simulink model "Follower_V2V"  (R2014b)
settings: Solver=ode3  SolverMode=SingleTasking  StartTime=0.0  StopTime=10.0  FixedStep=sampleTimes.main  RelTol=1e-3
model workspace (MAT data in the model file):
  spacing = 0
  vehicle = 0
undefined symbols (not defined in the file or in its folder): delays, sampleTimes
libraries: simulink x15
settings Model: ParameterArgumentNames=vehicle,spacing  Creator=uos  LastModifiedBy=uos

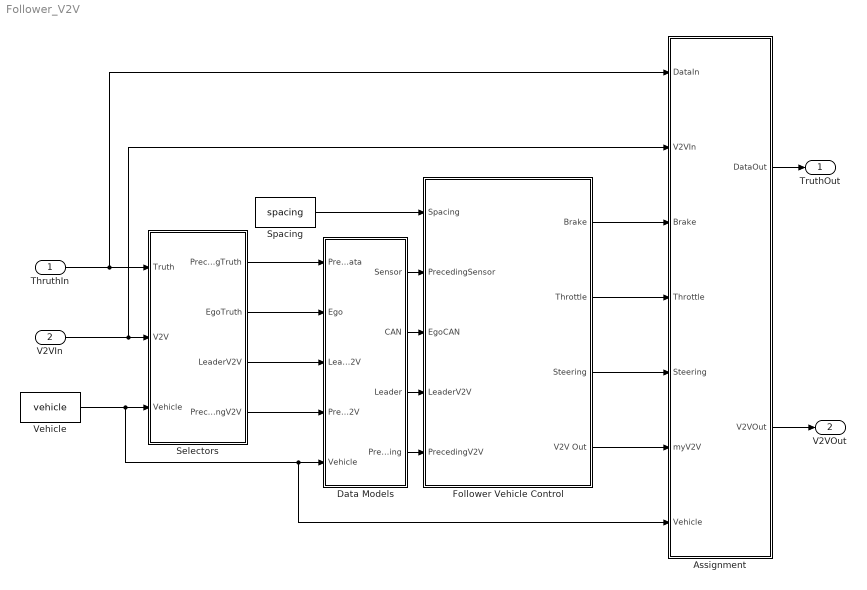
== system Follower_V2V ==
  ThruthIn : Inport  OutDataTypeStr=Bus: VehicleBus  PortDimensions=10  BusOutputAsStruct=on
  V2VIn : Inport  Port=2  OutDataTypeStr=Bus: V2VBus  PortDimensions=10  SampleTime=0  BusOutputAsStruct=on
  Assignment : Subsystem
  Data Models : Subsystem
  Follower Vehicle Control : Subsystem
  Selectors : Subsystem
  Spacing : Constant  Value=spacing
  Vehicle : Constant  Value=vehicle
  TruthOut : Outport  OutDataTypeStr=Bus: VehicleBus  PortDimensions=10  BusOutputAsStruct=on
  V2VOut : Outport  Port=2  OutDataTypeStr=Bus: V2VBus  PortDimensions=10  BusOutputAsStruct=on
  wires:
  ThruthIn/1 -> Assignment/1(DataIn), Selectors/1(Truth)
  Assignment/1(DataOut) -> TruthOut/1
  Spacing/1 -> Follower Vehicle Control/1(Spacing)
  Vehicle/1 -> Assignment/7(Vehicle), Data Models/5(Vehicle), Selectors/3(Vehicle)
  Follower Vehicle Control/1(Brake) -> Assignment/3(Brake)
  Follower Vehicle Control/2(Throttle) -> Assignment/4(Throttle)
  Follower Vehicle Control/3(Steering) -> Assignment/5(Steering)
  V2VIn/1 -> Assignment/2(V2VIn), Selectors/2(V2V)
  Assignment/2(V2VOut) -> V2VOut/1
  Follower Vehicle Control/4(V2V Out) -> Assignment/6(myV2V)
  Selectors/1(PrecedingTruth) -> Data Models/1(PrecedingData)
  Selectors/2(EgoTruth) -> Data Models/2(Ego)
  Selectors/3(LeaderV2V) -> Data Models/3(LeaderV2V)
  Selectors/4(PrecedingV2V) -> Data Models/4(PrecedingV2V)
  Data Models/1(Sensor) -> Follower Vehicle Control/2(PrecedingSensor)
  Data Models/2(CAN) -> Follower Vehicle Control/3(EgoCAN)
  Data Models/3(Leader) -> Follower Vehicle Control/4(LeaderV2V)
  Data Models/4(Preceding) -> Follower Vehicle Control/5(PrecedingV2V)

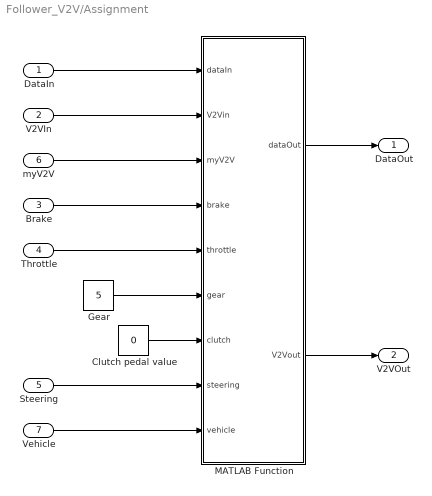
== system Follower_V2V/Assignment ==
  DataIn : Inport
  V2VIn : Inport  Port=2
  Brake : Inport  Port=3
  Throttle : Inport  Port=4
  Steering : Inport  Port=5
  myV2V : Inport  Port=6
  Vehicle : Inport  Port=7
  Clutch pedal value : Constant  Value=0
  Gear : Constant  Value=5  OutDataTypeStr=int32
  MATLAB Function : MATLAB Function  TreatAsAtomicUnit=on
  DataOut : Outport
  V2VOut : Outport  Port=2
  wires:
  Vehicle/1 -> MATLAB Function/9(vehicle)
  DataIn/1 -> MATLAB Function/1(dataIn)
  Brake/1 -> MATLAB Function/4(brake)
  MATLAB Function/1(dataOut) -> DataOut/1
  Throttle/1 -> MATLAB Function/5(throttle)
  Steering/1 -> MATLAB Function/8(steering)
  V2VIn/1 -> MATLAB Function/2(V2Vin)
  myV2V/1 -> MATLAB Function/3(myV2V)
  MATLAB Function/2(V2Vout) -> V2VOut/1
  Gear/1 -> MATLAB Function/6(gear)
  Clutch pedal value/1 -> MATLAB Function/7(clutch)

== system Follower_V2V/Data Models ==
  PrecedingData : Inport
  Ego : Inport  Port=2
  LeaderV2V : Inport  Port=3
  PrecedingV2V : Inport  Port=4
  Vehicle : Inport  Port=5
  Comms Model : Subsystem
  Sensor Model : Subsystem
  Sensor : Outport
  CAN : Outport  Port=2
  Leader : Outport  Port=3
  Preceding : Outport  Port=4
  wires:
  Sensor Model/2(EgoCAN) -> CAN/1
  Sensor Model/1(PreceedingSensor) -> Sensor/1
  PrecedingData/1 -> Sensor Model/1(PrceedingData)
  Ego/1 -> Sensor Model/2(EgoData)
  LeaderV2V/1 -> Comms Model/1(LeaderV2VIn)
  PrecedingV2V/1 -> Comms Model/2(PrecedingV2VIn)
  Comms Model/1(LeaderV2V) -> Leader/1
  Comms Model/2(PrecedingV2V) -> Preceding/1
  Vehicle/1 -> Sensor Model/3(Vehicle), Comms Model/3(Vehicle)

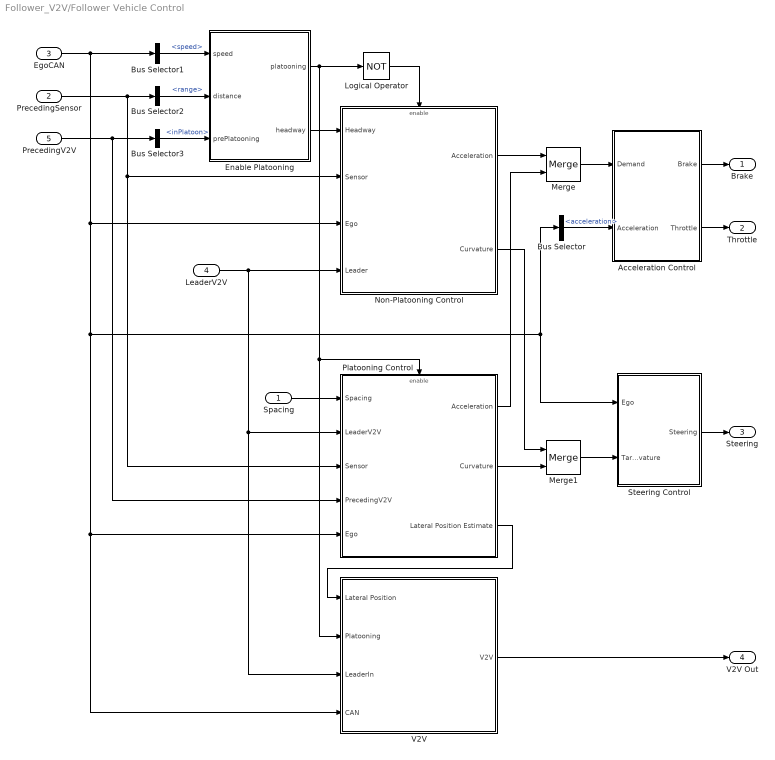
== system Follower_V2V/Follower Vehicle Control ==
  Spacing : Inport
  PrecedingSensor : Inport  Port=2
  EgoCAN : Inport  Port=3
  LeaderV2V : Inport  Port=4
  PrecedingV2V : Inport  Port=5
  Acceleration Control : Subsystem
  Bus Selector : BusSelector  OutputSignals=acceleration
  Bus Selector1 : BusSelector  OutputSignals=speed
  Bus Selector2 : BusSelector  OutputSignals=range
  Bus Selector3 : BusSelector  OutputSignals=inPlatoon
  Enable Platooning : Stateflow chart  TreatAsAtomicUnit=on
  Logical Operator : Logic  Operator=NOT  AllPortsSameDT=off  OutDataTypeStr=boolean
  Merge : Merge
  Merge1 : Merge
  Non-Platooning Control : Subsystem
  Platooning Control : Subsystem
  Steering Control : Subsystem
  V2V : Subsystem
  Brake : Outport
  Throttle : Outport  Port=2
  Steering : Outport  Port=3
  V2V Out : Outport  Port=4
  wires:
  Bus Selector/1 -> Acceleration Control/2(Acceleration)  "<acceleration>"
  Acceleration Control/1(Brake) -> Brake/1
  Acceleration Control/2(Throttle) -> Throttle/1
  Steering Control/1(Steering) -> Steering/1
  Spacing/1 -> Platooning Control/1(Spacing)
  LeaderV2V/1 -> Non-Platooning Control/4(Leader), V2V/3(LeaderIn), Platooning Control/2(LeaderV2V)
  PrecedingSensor/1 -> Platooning Control/3(Sensor), Non-Platooning Control/2(Sensor), Bus Selector2/1
  Merge/1 -> Acceleration Control/1(Demand)
  Platooning Control/1(Acceleration) -> Merge/2
  Non-Platooning Control/1(Acceleration) -> Merge/1
  Platooning Control/2(Curvature) -> Merge1/2
  Non-Platooning Control/2(Curvature) -> Merge1/1
  Enable Platooning/1(platooning) -> V2V/2(Platooning), Platooning Control/Enable, Logical Operator/1
  Logical Operator/1 -> Non-Platooning Control/Enable
  Bus Selector1/1 -> Enable Platooning/1(speed)  "<speed>"
  Bus Selector2/1 -> Enable Platooning/2(distance)  "<range>"
  EgoCAN/1 -> Bus Selector1/1, Non-Platooning Control/3(Ego), V2V/4(CAN), Platooning Control/5(Ego), Steering Control/1(Ego), Bus Selector/1
  Merge1/1 -> Steering Control/2(Target Curvature)
  V2V/1(V2V) -> V2V Out/1
  Enable Platooning/2(headway) -> Non-Platooning Control/1(Headway)
  PrecedingV2V/1 -> Bus Selector3/1, Platooning Control/4(PrecedingV2V)
  Platooning Control/3(Lateral Position Estimate) -> V2V/1(Lateral Position)
  Bus Selector3/1 -> Enable Platooning/3(prePlatooning)  "<inPlatoon>"

== system Follower_V2V/Selectors ==
  Truth : Inport
  V2V : Inport  Port=2
  Vehicle : Inport  Port=3
  MATLAB Function : MATLAB Function  TreatAsAtomicUnit=on
  PrecedingTruth : Outport
  EgoTruth : Outport  Port=2
  LeaderV2V : Outport  Port=3
  PrecedingV2V : Outport  Port=4
  wires:
  Truth/1 -> MATLAB Function/1(data)
  Vehicle/1 -> MATLAB Function/3(vehicle)
  MATLAB Function/2(egoTruth) -> EgoTruth/1
  V2V/1 -> MATLAB Function/2(V2V)
  MATLAB Function/3(leaderV2V) -> LeaderV2V/1
  MATLAB Function/4(precedingV2V) -> PrecedingV2V/1
  MATLAB Function/1(precedingTruth) -> PrecedingTruth/1

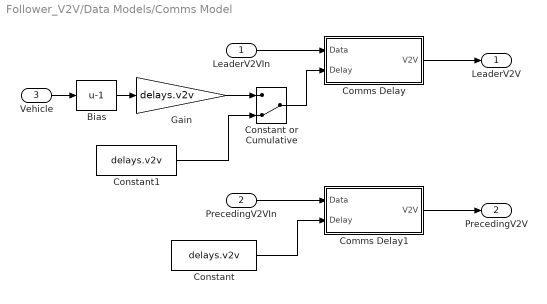
== system Follower_V2V/Data Models/Comms Model ==
  LeaderV2VIn : Inport
  PrecedingV2VIn : Inport  Port=2
  Vehicle : Inport  Port=3
  Bias : Bias  Bias=-1
  Comms Delay : Subsystem
  Comms Delay1 : Subsystem
  Constant : Constant  Value=delays.v2v
  Constant or Cumulative : ManualSwitch  CurrentSetting=0
  Constant1 : Constant  Value=delays.v2v
  Gain : Gain  Gain=delays.v2v
  LeaderV2V : Outport
  PrecedingV2V : Outport  Port=2
  wires:
  LeaderV2VIn/1 -> Comms Delay/1(Data)
  Comms Delay/1(V2V) -> LeaderV2V/1
  PrecedingV2VIn/1 -> Comms Delay1/1(Data)
  Comms Delay1/1(V2V) -> PrecedingV2V/1
  Constant/1 -> Comms Delay1/2(Delay)
  Constant or Cumulative/1 -> Comms Delay/2(Delay)
  Constant1/1 -> Constant or Cumulative/2
  Vehicle/1 -> Bias/1
  Bias/1 -> Gain/1
  Gain/1 -> Constant or Cumulative/1

== system Follower_V2V/Data Models/Sensor Model ==
  PrceedingData : Inport
  EgoData : Inport  Port=2
  Vehicle : Inport  Port=3
  CAN Model : Subsystem
  Radar Model : Subsystem
  PreceedingSensor : Outport
  EgoCAN : Outport  Port=2
  wires:
  EgoData/1 -> CAN Model/1(Data), Radar Model/2(Ego)
  Radar Model/1(Radar Data) -> PreceedingSensor/1
  CAN Model/1(CAN) -> EgoCAN/1
  PrceedingData/1 -> Radar Model/1(Target)
  Vehicle/1 -> CAN Model/2(Vehicle)

== system Follower_V2V/Follower Vehicle Control/Acceleration Control ==
  Demand : Inport
  Acceleration : Inport  Port=2
  Brake Control : Subsystem
  Compare To Constant : simulink/Logic and Bit Operations/Compare To Constant  relop=>=  const=-0.1  OutDataTypeStr=boolean
  Logical Operator : Logic  Operator=NOT  AllPortsSameDT=off  OutDataTypeStr=boolean
  Sum1 : Sum  Inputs=+-|
  Throttle Control : Subsystem
  Brake : Outport
  Throttle : Outport  Port=2
  wires:
  Acceleration/1 -> Throttle Control/2(Acceleration), Sum1/2
  Demand/1 -> Throttle Control/1(Demand), Compare To Constant/1, Sum1/1
  Sum1/1 -> Brake Control/1(Error)
  Brake Control/1(Brake) -> Brake/1
  Throttle Control/1(Throttle) -> Throttle/1
  Compare To Constant/1 -> Throttle Control/Enable, Logical Operator/1
  Logical Operator/1 -> Brake Control/Enable

== system Follower_V2V/Follower Vehicle Control/Non-Platooning Control ==
  Headway : Inport
  Sensor : Inport  Port=2
  Ego : Inport  Port=3
  Leader : Inport  Port=4
  Enable : EnablePort
  Speed Control : Subsystem
  Steering Control1 : Subsystem
  Acceleration : Outport
  Curvature : Outport  Port=2
  wires:
  Steering Control1/1(Target Curvature) -> Curvature/1
  Ego/1 -> Speed Control/2(Ego)
  Sensor/1 -> Steering Control1/1(Sensor), Speed Control/3(Leader)
  Headway/1 -> Speed Control/1(Headway)
  Speed Control/1(Acceleration Demand) -> Acceleration/1
  Leader/1 -> Steering Control1/2(Leader)

== system Follower_V2V/Follower Vehicle Control/Platooning Control ==
  Spacing : Inport
  LeaderV2V : Inport  Port=2
  Sensor : Inport  Port=3
  PrecedingV2V : Inport  Port=4
  Ego : Inport  Port=5
  Enable : EnablePort
  Speed Control : Subsystem
  Steering Control : Subsystem
  Acceleration : Outport
  Curvature : Outport  Port=2
  Lateral Position Estimate : Outport  Port=3
  wires:
  Speed Control/1(Acceleration Demand) -> Acceleration/1
  Spacing/1 -> Speed Control/1(Spacing)
  Sensor/1 -> Steering Control/4(Sensor), Speed Control/3(PreceedingSensor)
  LeaderV2V/1 -> Steering Control/3(Leader), Speed Control/2(LeaderV2V)
  PrecedingV2V/1 -> Steering Control/2(Preceeding), Speed Control/4(PreceedingV2V)
  Ego/1 -> Steering Control/1(Ego), Speed Control/5(Ego)
  Steering Control/1(Curvature Command) -> Curvature/1
  Steering Control/2(lateralError) -> Lateral Position Estimate/1

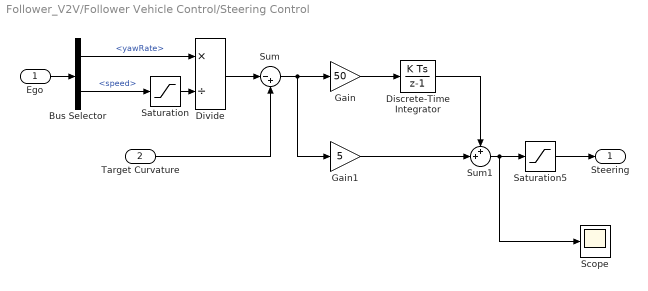
== system Follower_V2V/Follower Vehicle Control/Steering Control ==
  Ego : Inport
  Target Curvature : Inport  Port=2
  Bus Selector : BusSelector  OutputSignals=yawRate,speed
  Discrete-Time Integrator : DiscreteIntegrator  InitialCondition=0.0065  InitialConditionSetting=State (most efficient)  SampleTime=-1  LimitOutput=on  UpperSaturationLimit=0.5  LowerSaturationLimit=-0.5
  Divide : Product  Inputs=*/
  Gain : Gain  Gain=50
  Gain1 : Gain  Gain=5
  Saturation : Saturate  UpperLimit=inf  LowerLimit=1
  Saturation5 : Saturate
  Scope : Scope
  Sum : Sum  Inputs=|-+
  Sum1 : Sum  Inputs=++|
  Steering : Outport
  wires:
  Saturation5/1 -> Steering/1
  Sum1/1 -> Scope/1, Saturation5/1
  Target Curvature/1 -> Sum/2
  Ego/1 -> Bus Selector/1
  Bus Selector/2 -> Saturation/1  "<speed>"
  Bus Selector/1 -> Divide/1  "<yawRate>"
  Saturation/1 -> Divide/2
  Divide/1 -> Sum/1
  Gain/1 -> Discrete-Time Integrator/1
  Sum/1 -> Gain/1, Gain1/1
  Gain1/1 -> Sum1/2
  Discrete-Time Integrator/1 -> Sum1/1

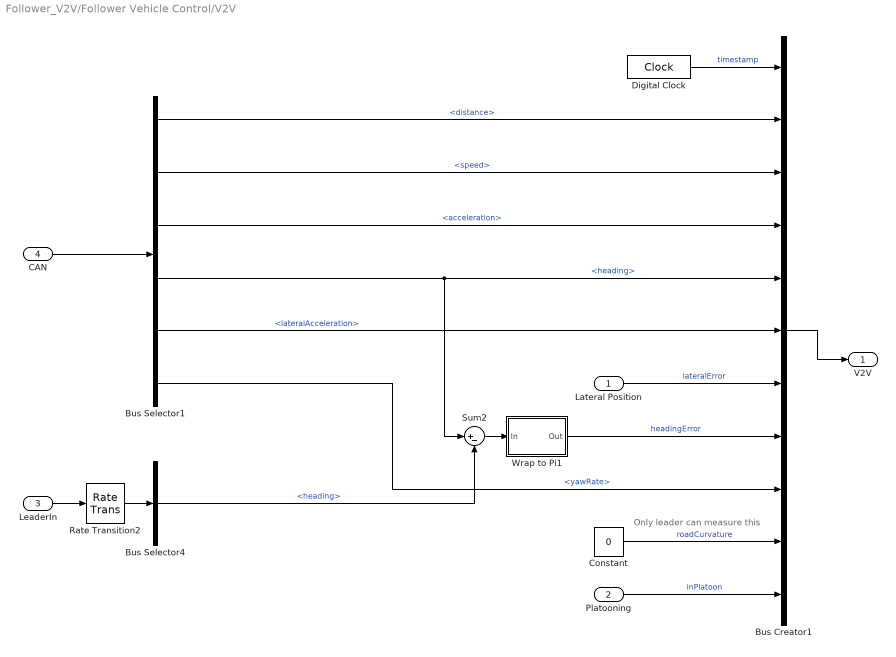
== system Follower_V2V/Follower Vehicle Control/V2V ==
  note: Only leader can measure this
  Lateral Position : Inport
  Platooning : Inport  Port=2
  LeaderIn : Inport  Port=3
  CAN : Inport  Port=4
  Bus Creator1 : BusCreator  Inputs=11  OutDataTypeStr=Bus: V2VBus  NonVirtualBus=on
  Bus Selector1 : BusSelector  OutputSignals=distance,speed,acceleration,heading,lateralAcceleration,yawRate
  Bus Selector4 : BusSelector  OutputSignals=heading
  Constant : Constant  Value=0
  Digital Clock : DigitalClock  SampleTime=sampleTimes.control
  Rate Transition2 : RateTransition  OutPortSampleTime=sampleTimes.control
  Sum2 : Sum  Inputs=|+-
  Wrap to Pi1 : Subsystem
  V2V : Outport
  wires:
  CAN/1 -> Bus Selector1/1
  Bus Selector1/6 -> Bus Creator1/9  "<yawRate>"
  Constant/1 -> Bus Creator1/10  "roadCurvature"
  Bus Selector1/3 -> Bus Creator1/4  "<acceleration>"
  Bus Selector1/1 -> Bus Creator1/2  "<distance>"
  Bus Selector1/2 -> Bus Creator1/3  "<speed>"
  Bus Selector1/5 -> Bus Creator1/6  "<lateralAcceleration>"
  Bus Creator1/1 -> V2V/1
  Bus Selector1/4 -> Bus Creator1/5, Sum2/1  "<heading>"
  Sum2/1 -> Wrap to Pi1/1(In)
  LeaderIn/1 -> Rate Transition2/1
  Rate Transition2/1 -> Bus Selector4/1
  Bus Selector4/1 -> Sum2/2  "<heading>"
  Wrap to Pi1/1(Out) -> Bus Creator1/8  "headingError"
  Lateral Position/1 -> Bus Creator1/7  "lateralError"
  Platooning/1 -> Bus Creator1/11  "inPlatoon"
  Digital Clock/1 -> Bus Creator1/1  "timestamp"

== system Follower_V2V/Data Models/Comms Model/Comms Delay ==
  Data : Inport
  Delay : Inport  Port=2
  Display : Display
  Rate Transition1 : RateTransition  OutPortSampleTime=sampleTimes.v2v
  Rate Transition2 : RateTransition  OutPortSampleTime=sampleTimes.main
  Variable Integer Delay : Delay  DelayLengthSource=Input port
      settings: InputPortMap=u0,p1
  Weighted Sample Time Math : SampleTimeMath  TsampMathOp=/
  V2V : Outport
  wires:
  Rate Transition1/1 -> V2V/1
  Data/1 -> Rate Transition2/1
  Rate Transition2/1 -> Variable Integer Delay/1
  Delay/1 -> Weighted Sample Time Math/1
  Weighted Sample Time Math/1 -> Display/1, Variable Integer Delay/2
  Variable Integer Delay/1 -> Rate Transition1/1

== system Follower_V2V/Data Models/Comms Model/Comms Delay1 ==
  Data : Inport
  Delay : Inport  Port=2
  Rate Transition1 : RateTransition  OutPortSampleTime=sampleTimes.v2v
  Rate Transition2 : RateTransition  OutPortSampleTime=sampleTimes.main
  Variable Integer Delay : Delay  DelayLengthSource=Input port
      settings: InputPortMap=u0,p1
  Weighted Sample Time Math : SampleTimeMath  TsampMathOp=/
  V2V : Outport
  wires:
  Variable Integer Delay/1 -> Rate Transition1/1
  Weighted Sample Time Math/1 -> Variable Integer Delay/2
  Delay/1 -> Weighted Sample Time Math/1
  Rate Transition2/1 -> Variable Integer Delay/1
  Data/1 -> Rate Transition2/1
  Rate Transition1/1 -> V2V/1

== system Follower_V2V/Data Models/Sensor Model/CAN Model ==
  Data : Inport
  Vehicle : Inport  Port=2
  Bus Creator : BusCreator  Inputs=7
  Bus Selector : BusSelector  OutputSignals=data.roadDistance,data.velocity,data.acceleration,data.angularVelocity,data.angle
  Gain : Gain
  Rate Transition1 : RateTransition  OutPortSampleTime=sampleTimes.main
  Selector : Selector  InputPortWidth=3
  Selector1 : Selector  InputPortWidth=3
  Selector2 : Selector  InputPortWidth=3  Indices=3
  Selector3 : Selector  InputPortWidth=3  Indices=2
  Selector4 : Selector  InputPortWidth=3  Indices=3
  CAN : Outport
  wires:
  Rate Transition1/1 -> CAN/1
  Bus Creator/1 -> Rate Transition1/1
  Selector1/1 -> Bus Creator/3  "acceleration"
  Bus Selector/3 -> Selector1/1, Selector3/1  "<acceleration>"
  Selector/1 -> Bus Creator/2  "speed"
  Bus Selector/2 -> Selector/1  "<velocity>"
  Data/1 -> Bus Selector/1
  Bus Selector/4 -> Selector2/1  "<angularVelocity>"
  Selector2/1 -> Bus Creator/5  "yawRate"
  Selector3/1 -> Bus Creator/4  "lateralAcceleration"
  Bus Selector/5 -> Selector4/1  "<angle>"
  Selector4/1 -> Bus Creator/6  "heading"
  Bus Selector/1 -> Gain/1  "<roadDistance>"
  Gain/1 -> Bus Creator/1  "distance"
  Vehicle/1 -> Bus Creator/7  "vehicle"

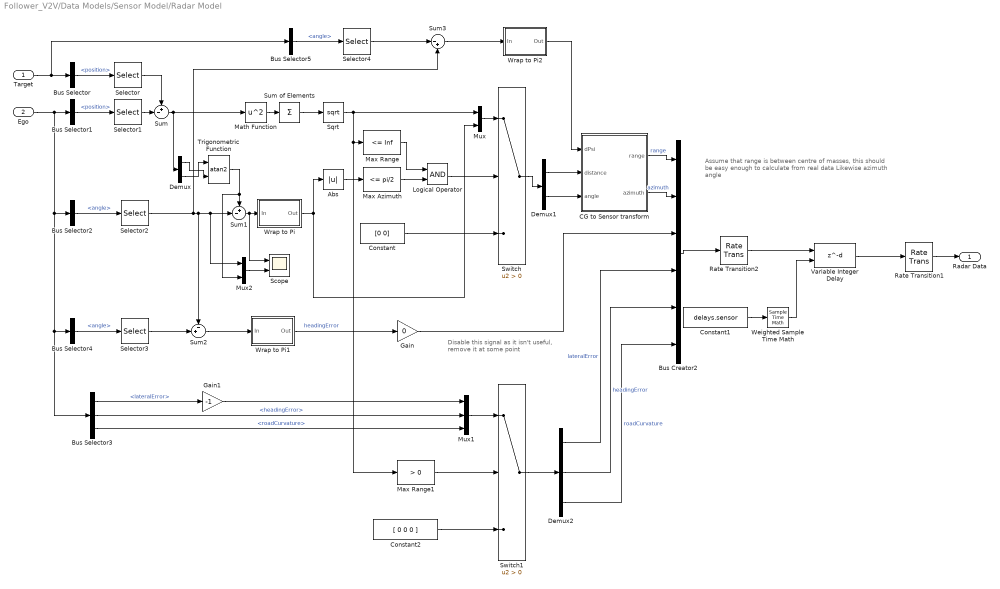
== system Follower_V2V/Data Models/Sensor Model/Radar Model ==
  note: Assume that range is between centre of masses,
      | this should be easy enough to calculate from real data
      | Likewise azimuth angle
  note: Disable this signal as it isn't useful,
      | remove it at some point
  Target : Inport
  Ego : Inport  Port=2
  Abs : Abs
  Bus Creator2 : BusCreator  Inputs=6
  Bus Selector : BusSelector  OutputSignals=data.position
  Bus Selector1 : BusSelector  OutputSignals=data.position
  Bus Selector2 : BusSelector  OutputSignals=data.angle
  Bus Selector3 : BusSelector  OutputSignals=data.lateralError,data.headingError,data.roadCurvature
  Bus Selector4 : BusSelector  OutputSignals=data.angle
  Bus Selector5 : BusSelector  OutputSignals=data.angle
  CG to Sensor transform : Subsystem
  Constant : Constant  Value=[0 0]
  Constant1 : Constant  Value=delays.sensor
  Constant2 : Constant  Value=[ 0 0 0 ]
  Demux : Demux  Outputs=2
  Demux1 : Demux  Outputs=2
  Demux2 : Demux  Outputs=3
  Gain : Gain  Gain=0
  Gain1 : Gain  Gain=-1
  Logical Operator : Logic  AllPortsSameDT=off  OutDataTypeStr=boolean
  Math Function : Math  Operator=square  SaturateOnIntegerOverflow=on
  Max Azimuth : simulink/Logic and Bit Operations/Compare To Constant  relop=<=  const=pi/2  OutDataTypeStr=boolean
  Max Range : simulink/Logic and Bit Operations/Compare To Constant  relop=<=  const=Inf  OutDataTypeStr=boolean
  Max Range1 : simulink/Logic and Bit Operations/Compare To Constant  relop=>  const=0  OutDataTypeStr=boolean
  Mux : Mux  Inputs=2
  Mux1 : Mux  Inputs=3
  Mux2 : Mux  Inputs=2
  Rate Transition1 : RateTransition  OutPortSampleTime=sampleTimes.sensor
  Rate Transition2 : RateTransition  OutPortSampleTime=sampleTimes.main
  Scope : Scope  NumInputPorts=2
      settings: YMin=-5~-5  YMax=5~5  SaveName=ScopeData11
  Selector : Selector  InputPortWidth=3  Indices=[1 2]
  Selector1 : Selector  InputPortWidth=3  Indices=[1 2]
  Selector2 : Selector  InputPortWidth=3  Indices=3
  Selector3 : Selector  InputPortWidth=3  Indices=3
  Selector4 : Selector  InputPortWidth=3  Indices=3
  Sqrt : Sqrt  SaturateOnIntegerOverflow=on
  Sum : Sum  Inputs=+-|
  Sum of Elements : Sum  Inputs=+
  Sum1 : Sum  Inputs=+-|
  Sum2 : Sum  Inputs=-+|
  Sum3 : Sum  Inputs=|-+
  Switch : Switch  Criteria=u2 > Threshold
  Switch1 : Switch  Criteria=u2 > Threshold
  Trigonometric Function : Trigonometry  Operator=atan2
  Variable Integer Delay : Delay  DelayLengthSource=Input port
      settings: InputPortMap=u0,p1
  Weighted Sample Time Math : SampleTimeMath  TsampMathOp=/
  Wrap to Pi : Subsystem
  Wrap to Pi1 : Subsystem
  Wrap to Pi2 : Subsystem
  Radar Data : Outport
  wires:
  Selector1/1 -> Sum/2
  Selector/1 -> Sum/1
  Bus Selector/1 -> Selector/1  "<position>"
  Bus Selector1/1 -> Selector1/1  "<position>"
  Bus Selector2/1 -> Selector2/1  "<angle>"
  Sum/1 -> Math Function/1, Demux/1
  Selector2/1 -> Sum2/1, Mux2/1, Sum1/2, Sum3/2
  Trigonometric Function/1 -> Mux2/2, Sum1/1
  Sum1/1 -> Scope/1, Wrap to Pi/1(In)
  Math Function/1 -> Sum of Elements/1
  Sum of Elements/1 -> Sqrt/1
  Constant/1 -> Switch/3
  Logical Operator/1 -> Switch/2
  Max Range/1 -> Logical Operator/1
  Abs/1 -> Max Azimuth/1
  Max Azimuth/1 -> Logical Operator/2
  Demux/1 -> Trigonometric Function/2
  Demux/2 -> Trigonometric Function/1
  Wrap to Pi/1(Out) -> Mux/2, Abs/1
  Bus Creator2/1 -> Rate Transition2/1
  Rate Transition1/1 -> Radar Data/1
  Rate Transition2/1 -> Variable Integer Delay/1
  Variable Integer Delay/1 -> Rate Transition1/1
  Constant1/1 -> Weighted Sample Time Math/1
  Weighted Sample Time Math/1 -> Variable Integer Delay/2
  Bus Selector4/1 -> Selector3/1  "<angle>"
  Selector3/1 -> Sum2/2
  Sum2/1 -> Wrap to Pi1/1(In)
  Demux1/2 -> CG to Sensor transform/3(angle)
  Mux/1 -> Switch/1
  Sqrt/1 -> Mux/1, Max Range1/1, Max Range/1
  Switch/1 -> Demux1/1
  Wrap to Pi1/1(Out) -> Gain/1  "headingError"
  Gain/1 -> Bus Creator2/3
  Ego/1 -> Bus Selector2/1, Bus Selector3/1, Bus Selector4/1, Bus Selector1/1
  Mux1/1 -> Switch1/1
  Bus Selector3/1 -> Gain1/1  "<lateralError>"
  Bus Selector3/2 -> Mux1/2  "<headingError>"
  Max Range1/1 -> Switch1/2
  Constant2/1 -> Switch1/3
  Switch1/1 -> Demux2/1
  Demux2/1 -> Bus Creator2/4  "lateralError"
  Demux2/2 -> Bus Creator2/5  "headingError"
  Bus Selector3/3 -> Mux1/3  "<roadCurvature>"
  Demux2/3 -> Bus Creator2/6  "roadCurvature"
  Mux2/1 -> Scope/2
  Gain1/1 -> Mux1/1
  Bus Selector5/1 -> Selector4/1  "<angle>"
  Target/1 -> Bus Selector5/1, Bus Selector/1
  Selector4/1 -> Sum3/1
  Sum3/1 -> Wrap to Pi2/1(In)
  Wrap to Pi2/1(Out) -> CG to Sensor transform/1(dPsi)
  CG to Sensor transform/1(range) -> Bus Creator2/1  "range"
  CG to Sensor transform/2(azimuth) -> Bus Creator2/2  "azimuth"
  Demux1/1 -> CG to Sensor transform/2(distance)

== system Follower_V2V/Follower Vehicle Control/Acceleration Control/Brake Control ==
  Error : Inport
  Enable : EnablePort  StatesWhenEnabling=reset
  Discrete-Time Integrator : DiscreteIntegrator  InitialConditionSetting=State (most efficient)  SampleTime=-1  LimitOutput=on  UpperSaturationLimit=1  LowerSaturationLimit=-1
  Gain2 : Gain  Gain=0.005
  Gain3 : Gain
  Saturation1 : Saturate  UpperLimit=1  LowerLimit=0
  Sum2 : Sum  Inputs=++|
  Unary Minus : UnaryMinus
  Brake : Outport  OutputWhenDisabled=reset  InitialOutput=0
  wires:
  Saturation1/1 -> Brake/1
  Sum2/1 -> Saturation1/1
  Error/1 -> Unary Minus/1
  Gain2/1 -> Sum2/2
  Discrete-Time Integrator/1 -> Sum2/1
  Gain3/1 -> Discrete-Time Integrator/1
  Unary Minus/1 -> Gain2/1, Gain3/1

== system Follower_V2V/Follower Vehicle Control/Acceleration Control/Throttle Control ==
  Demand : Inport
  Acceleration : Inport  Port=2
  Enable : EnablePort  StatesWhenEnabling=reset
  Discrete-Time Integrator : DiscreteIntegrator  InitialConditionSetting=State (most efficient)  SampleTime=-1  LimitOutput=on  UpperSaturationLimit=1  LowerSaturationLimit=-1
  Gain : Gain  Gain=1.5
  Gain1 : Gain  Gain=10
  Sum : Sum  Inputs=++|
  Sum1 : Sum  Inputs=+-|
  Throttle : Outport  OutputWhenDisabled=reset  InitialOutput=0
  wires:
  Gain/1 -> Sum/1
  Discrete-Time Integrator/1 -> Sum/2
  Gain1/1 -> Discrete-Time Integrator/1
  Sum/1 -> Throttle/1
  Demand/1 -> Sum1/1, Gain/1
  Acceleration/1 -> Sum1/2
  Sum1/1 -> Gain1/1

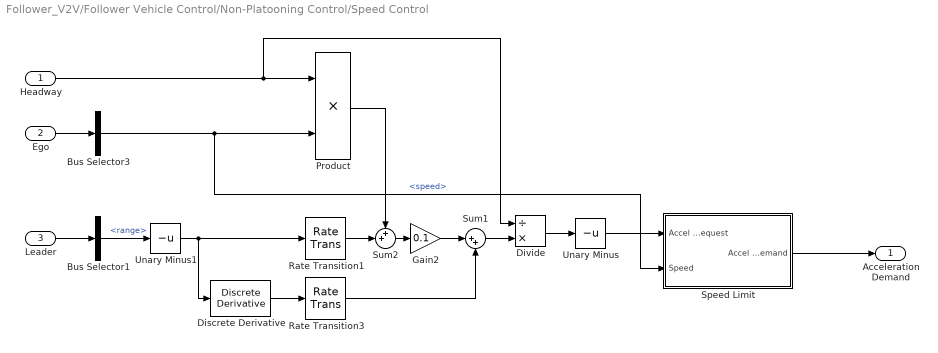
== system Follower_V2V/Follower Vehicle Control/Non-Platooning Control/Speed Control ==
  Headway : Inport
  Ego : Inport  Port=2
  Leader : Inport  Port=3
  Bus Selector1 : BusSelector  OutputSignals=range
  Bus Selector3 : BusSelector  OutputSignals=speed
  Discrete Derivative : simulink/Discrete/Discrete Derivative  gainval=1.0  ICPrevScaledInput=0.0  InputProcessing=Inherited  OutMin=[]  OutMax=[]  OutDataType=fixdt(1, 16)  OutScaling=2^-10  DoSatur=off
  Divide : Product  Inputs=/*
  Gain2 : Gain  Gain=0.1
  Product : Product
  Rate Transition1 : RateTransition  OutPortSampleTime=sampleTimes.control
  Rate Transition3 : RateTransition  OutPortSampleTime=sampleTimes.control
  Speed Limit : Subsystem
  Sum1 : Sum  Inputs=|++
  Sum2 : Sum  Inputs=++|
  Unary Minus : UnaryMinus
  Unary Minus1 : UnaryMinus
  Acceleration Demand : Outport
  wires:
  Ego/1 -> Bus Selector3/1
  Leader/1 -> Bus Selector1/1
  Bus Selector3/1 -> Speed Limit/2(Speed), Product/2  "<speed>"
  Headway/1 -> Divide/1, Product/1
  Bus Selector1/1 -> Unary Minus1/1  "<range>"
  Product/1 -> Sum2/1
  Sum2/1 -> Gain2/1
  Gain2/1 -> Sum1/1
  Discrete Derivative/1 -> Rate Transition3/1
  Sum1/1 -> Divide/2
  Divide/1 -> Unary Minus/1
  Unary Minus/1 -> Speed Limit/1(Accel Request)
  Rate Transition3/1 -> Sum1/2
  Rate Transition1/1 -> Sum2/2
  Unary Minus1/1 -> Discrete Derivative/1, Rate Transition1/1
  Speed Limit/1(Accel Demand) -> Acceleration Demand/1

== system Follower_V2V/Follower Vehicle Control/Non-Platooning Control/Steering Control1 ==
  note: Uses the understeer gradient relationship
      | Future work could include learning the gardient as it appears to have a weak dependence on speed
  note: Lateral controller based on curvature
  Sensor : Inport
  Leader : Inport  Port=2
  Add2 : Sum  Inputs=+++
  Bus Selector1 : BusSelector  OutputSignals=headingError,lateralError,roadCurvature
  Bus Selector2 : BusSelector  OutputSignals=lateralError
  Sum : Sum  Inputs=|+-
  kh : Gain  Gain=0.05
  ky : Gain  Gain=0.00075
  Target Curvature : Outport
  wires:
  Sum/1 -> ky/1
  kh/1 -> Add2/1
  ky/1 -> Add2/2
  Add2/1 -> Target Curvature/1
  Sensor/1 -> Bus Selector1/1
  Bus Selector1/1 -> kh/1  "<headingError>"
  Bus Selector1/3 -> Add2/3  "<roadCurvature>"
  Leader/1 -> Bus Selector2/1
  Bus Selector2/1 -> Sum/2  "<lateralError>"
  Bus Selector1/2 -> Sum/1  "<lateralError>"

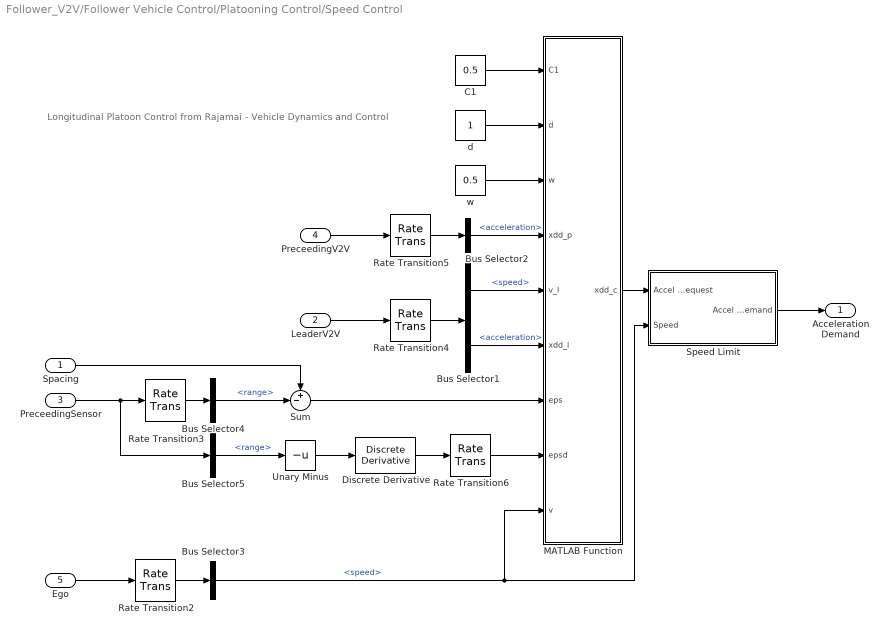
== system Follower_V2V/Follower Vehicle Control/Platooning Control/Speed Control ==
  note: Longitudinal Platoon Control from Rajamai - Vehicle Dynamics and Control
  Spacing : Inport
  LeaderV2V : Inport  Port=2
  PreceedingSensor : Inport  Port=3
  PreceedingV2V : Inport  Port=4
  Ego : Inport  Port=5
  Bus Selector1 : BusSelector  OutputSignals=speed,acceleration
  Bus Selector2 : BusSelector  OutputSignals=acceleration
  Bus Selector3 : BusSelector  OutputSignals=speed
  Bus Selector4 : BusSelector  OutputSignals=range
  Bus Selector5 : BusSelector  OutputSignals=range
  C1 : Constant  Value=0.5
  Discrete Derivative : simulink/Discrete/Discrete Derivative  gainval=1.0  ICPrevScaledInput=0.0  InputProcessing=Inherited  OutMin=[]  OutMax=[]  OutDataType=fixdt(1, 16)  OutScaling=2^-10  DoSatur=off
  MATLAB Function : MATLAB Function  TreatAsAtomicUnit=on
  Rate Transition2 : RateTransition  OutPortSampleTime=sampleTimes.control
  Rate Transition3 : RateTransition  OutPortSampleTime=sampleTimes.control
  Rate Transition4 : RateTransition  Deterministic=off  OutPortSampleTime=sampleTimes.control
  Rate Transition5 : RateTransition  Deterministic=off  OutPortSampleTime=sampleTimes.control
  Rate Transition6 : RateTransition  Deterministic=off  OutPortSampleTime=sampleTimes.control
  Speed Limit : Subsystem
  Sum : Sum  Inputs=+-|
  Unary Minus : UnaryMinus
  d : Constant
  w : Constant  Value=0.5
  Acceleration Demand : Outport
  wires:
  Ego/1 -> Rate Transition2/1
  Bus Selector3/1 -> Speed Limit/2(Speed), MATLAB Function/9(v)  "<speed>"
  PreceedingSensor/1 -> Bus Selector5/1, Rate Transition3/1
  Bus Selector4/1 -> Sum/2  "<range>"
  Discrete Derivative/1 -> Rate Transition6/1
  Speed Limit/1(Accel Demand) -> Acceleration Demand/1
  C1/1 -> MATLAB Function/1(C1)
  d/1 -> MATLAB Function/2(d)
  w/1 -> MATLAB Function/3(w)
  Spacing/1 -> Sum/1
  LeaderV2V/1 -> Rate Transition4/1
  Bus Selector1/2 -> MATLAB Function/6(xdd_l)  "<acceleration>"
  Bus Selector1/1 -> MATLAB Function/5(v_l)  "<speed>"
  PreceedingV2V/1 -> Rate Transition5/1
  Bus Selector2/1 -> MATLAB Function/4(xdd_p)  "<acceleration>"
  Rate Transition2/1 -> Bus Selector3/1
  Rate Transition3/1 -> Bus Selector4/1
  Rate Transition4/1 -> Bus Selector1/1
  Rate Transition5/1 -> Bus Selector2/1
  Bus Selector5/1 -> Unary Minus/1  "<range>"
  Rate Transition6/1 -> MATLAB Function/8(epsd)
  Sum/1 -> MATLAB Function/7(eps)
  Unary Minus/1 -> Discrete Derivative/1
  MATLAB Function/1(xdd_c) -> Speed Limit/1(Accel Request)

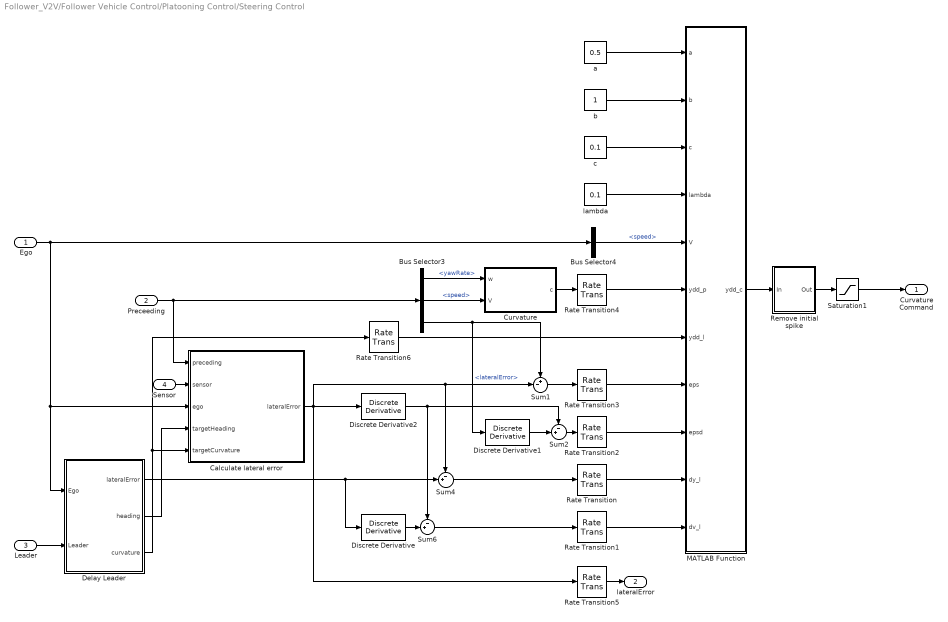
== system Follower_V2V/Follower Vehicle Control/Platooning Control/Steering Control ==
  Ego : Inport
  Preceeding : Inport  Port=2
  Leader : Inport  Port=3
  Sensor : Inport  Port=4
  Bus Selector3 : BusSelector  OutputSignals=yawRate,speed,lateralError
  Bus Selector4 : BusSelector  OutputSignals=speed
  Calculate lateral error : Subsystem
  Curvature : MATLAB Function  TreatAsAtomicUnit=on
  Delay Leader : Subsystem
  Discrete Derivative : simulink/Discrete/Discrete Derivative  gainval=1.0  ICPrevScaledInput=0.0  InputProcessing=Inherited  OutMin=[]  OutMax=[]  OutDataType=fixdt(1, 16)  OutScaling=2^-10  DoSatur=off
  Discrete Derivative1 : simulink/Discrete/Discrete Derivative  gainval=1.0  ICPrevScaledInput=0.0  InputProcessing=Inherited  OutMin=[]  OutMax=[]  OutDataType=fixdt(1, 16)  OutScaling=2^-10  DoSatur=off
  Discrete Derivative2 : simulink/Discrete/Discrete Derivative  gainval=1.0  ICPrevScaledInput=0.0  InputProcessing=Inherited  OutMin=[]  OutMax=[]  OutDataType=fixdt(1, 16)  OutScaling=2^-10  DoSatur=off
  MATLAB Function : MATLAB Function  TreatAsAtomicUnit=on
  Rate Transition : RateTransition  Integrity=off  Deterministic=off  OutPortSampleTime=sampleTimes.control
  Rate Transition{1..4,6} (5 alike) : RateTransition  OutPortSampleTime=sampleTimes.control
  Rate Transition5 : RateTransition  Integrity=off  Deterministic=off  OutPortSampleTime=sampleTimes.control
  Remove initial spike : Subsystem
  Saturation1 : Saturate  UpperLimit=0.1  LowerLimit=-0.1
  Sum1 : Sum  Inputs=+-|
  Sum2 : Sum  Inputs=-+|
  Sum4 : Sum  Inputs=-+|
  Sum6 : Sum  Inputs=-+|
  a : Constant  Value=0.5
  b : Constant
  c : Constant  Value=0.1
  lambda : Constant  Value=0.1
  Curvature Command : Outport
  lateralError : Outport  Port=2
  wires:
  Curvature/1(c) -> Rate Transition4/1
  Rate Transition/1 -> MATLAB Function/10(dy_l)
  Delay Leader/2(heading) -> Calculate lateral error/4(targetHeading)
  Sum6/1 -> Rate Transition1/1
  Rate Transition1/1 -> MATLAB Function/11(dv_l)
  Leader/1 -> Delay Leader/2(Leader)
  Sum4/1 -> Rate Transition/1
  Preceeding/1 -> Bus Selector3/1, Calculate lateral error/1(preceding)
  Rate Transition2/1 -> MATLAB Function/9(epsd)
  Rate Transition4/1 -> MATLAB Function/6(ydd_p)
  c/1 -> MATLAB Function/3(c)
  b/1 -> MATLAB Function/2(b)
  a/1 -> MATLAB Function/1(a)
  Saturation1/1 -> Curvature Command/1
  Sensor/1 -> Calculate lateral error/2(sensor)
  lambda/1 -> MATLAB Function/4(lambda)
  Bus Selector4/1 -> MATLAB Function/5(V)  "<speed>"
  Rate Transition5/1 -> lateralError/1
  Delay Leader/1(lateralError) -> Sum4/2, Discrete Derivative/1
  Ego/1 -> Bus Selector4/1, Delay Leader/1(Ego), Calculate lateral error/3(ego)
  Rate Transition3/1 -> MATLAB Function/8(eps)
  Bus Selector3/3 -> Discrete Derivative1/1, Sum1/1  "<lateralError>"
  Bus Selector3/2 -> Curvature/2(V)  "<speed>"
  Bus Selector3/1 -> Curvature/1(w)  "<yawRate>"
  Delay Leader/3(curvature) -> Rate Transition6/1, Calculate lateral error/5(targetCurvature)
  Rate Transition6/1 -> MATLAB Function/7(ydd_l)
  Sum2/1 -> Rate Transition2/1
  Sum1/1 -> Rate Transition3/1
  Calculate lateral error/1(lateralError) -> Sum4/1, Sum1/2, Rate Transition5/1, Discrete Derivative2/1
  MATLAB Function/1(ydd_c) -> Remove initial spike/1(In)
  Remove initial spike/1(Out) -> Saturation1/1
  Discrete Derivative1/1 -> Sum2/2
  Discrete Derivative/1 -> Sum6/2
  Discrete Derivative2/1 -> Sum6/1, Sum2/1

== system Follower_V2V/Follower Vehicle Control/V2V/Wrap to Pi1 ==
  In : Inport
  Bias : Bias  Bias=pi
  Bias1 : Bias  Bias=-pi
  Constant : Constant  Value=2*pi
  Math Function : Math  Operator=mod  SaturateOnIntegerOverflow=on
  Out : Outport
  wires:
  Constant/1 -> Math Function/2
  Bias1/1 -> Out/1
  Math Function/1 -> Bias1/1
  Bias/1 -> Math Function/1
  In/1 -> Bias/1

== system Follower_V2V/Data Models/Sensor Model/Radar Model/CG to Sensor transform ==
  dPsi : Inport
  distance : Inport  Port=2
  angle : Inport  Port=3
  MATLAB Function : MATLAB Function  TreatAsAtomicUnit=on
  range : Outport
  azimuth : Outport  Port=2
  wires:
  distance/1 -> MATLAB Function/1(d)
  angle/1 -> MATLAB Function/2(theta)
  dPsi/1 -> MATLAB Function/3(dpsi)
  MATLAB Function/1(d_r) -> range/1
  MATLAB Function/2(theta_c) -> azimuth/1

== system Follower_V2V/Data Models/Sensor Model/Radar Model/Wrap to Pi ==
  In : Inport
  Bias : Bias  Bias=pi
  Bias1 : Bias  Bias=-pi
  Constant : Constant  Value=2*pi
  Math Function : Math  Operator=mod  SaturateOnIntegerOverflow=on
  Out : Outport
  wires:
  In/1 -> Bias/1
  Bias/1 -> Math Function/1
  Math Function/1 -> Bias1/1
  Bias1/1 -> Out/1
  Constant/1 -> Math Function/2

== system Follower_V2V/Data Models/Sensor Model/Radar Model/Wrap to Pi1 ==
  In : Inport
  Bias : Bias  Bias=pi
  Bias1 : Bias  Bias=-pi
  Constant : Constant  Value=2*pi
  Math Function : Math  Operator=mod  SaturateOnIntegerOverflow=on
  Out : Outport
  wires:
  Constant/1 -> Math Function/2
  Bias1/1 -> Out/1
  Math Function/1 -> Bias1/1
  Bias/1 -> Math Function/1
  In/1 -> Bias/1

== system Follower_V2V/Data Models/Sensor Model/Radar Model/Wrap to Pi2 ==
  In : Inport
  Bias : Bias  Bias=pi
  Bias1 : Bias  Bias=-pi
  Constant : Constant  Value=2*pi
  Math Function : Math  Operator=mod  SaturateOnIntegerOverflow=on
  Out : Outport
  wires:
  Constant/1 -> Math Function/2
  Bias1/1 -> Out/1
  Math Function/1 -> Bias1/1
  Bias/1 -> Math Function/1
  In/1 -> Bias/1

== system Follower_V2V/Follower Vehicle Control/Non-Platooning Control/Speed Control/Speed Limit ==
  Accel Request : Inport
  Speed : Inport  Port=2
  70mph : simulink/Logic and Bit Operations/Compare To Constant  relop=<  const=31.3  OutDataTypeStr=boolean
  Compare To Zero : simulink/Logic and Bit Operations/Compare To Zero  relop=<  OutDataTypeStr=boolean
  Constant3 : Constant  Value=0
  Logical Operator : Logic  Operator=OR  AllPortsSameDT=off  OutDataTypeStr=boolean
  Switch : Switch  Criteria=u2 > Threshold
  Accel Demand : Outport
  wires:
  Speed/1 -> 70mph/1
  Compare To Zero/1 -> Logical Operator/1
  Logical Operator/1 -> Switch/2
  70mph/1 -> Logical Operator/2
  Constant3/1 -> Switch/3
  Accel Request/1 -> Compare To Zero/1, Switch/1
  Switch/1 -> Accel Demand/1

== system Follower_V2V/Follower Vehicle Control/Platooning Control/Speed Control/Speed Limit ==
  Accel Request : Inport
  Speed : Inport  Port=2
  70mph : simulink/Logic and Bit Operations/Compare To Constant  relop=<  const=31.3  OutDataTypeStr=boolean
  Compare To Zero : simulink/Logic and Bit Operations/Compare To Zero  relop=<  OutDataTypeStr=boolean
  Constant3 : Constant  Value=0
  Logical Operator : Logic  Operator=OR  AllPortsSameDT=off  OutDataTypeStr=boolean
  Switch : Switch  Criteria=u2 > Threshold
  Accel Demand : Outport
  wires:
  Speed/1 -> 70mph/1
  Compare To Zero/1 -> Logical Operator/1
  Logical Operator/1 -> Switch/2
  70mph/1 -> Logical Operator/2
  Constant3/1 -> Switch/3
  Accel Request/1 -> Compare To Zero/1, Switch/1
  Switch/1 -> Accel Demand/1

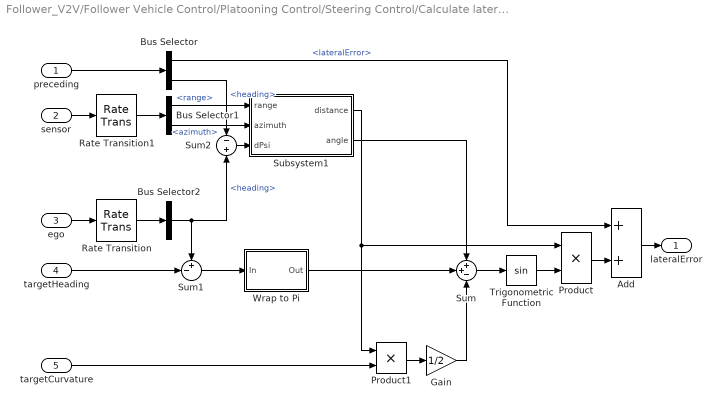
== system Follower_V2V/Follower Vehicle Control/Platooning Control/Steering Control/Calculate lateral error ==
  preceding : Inport
  sensor : Inport  Port=2
  ego : Inport  Port=3
  targetHeading : Inport  Port=4
  targetCurvature : Inport  Port=5
  Add : Sum
  Bus Selector : BusSelector  OutputSignals=lateralError,heading
  Bus Selector1 : BusSelector  OutputSignals=range,azimuth
  Bus Selector2 : BusSelector  OutputSignals=heading
  Gain : Gain  Gain=1/2
  Product : Product
  Product1 : Product
  Rate Transition : RateTransition  Integrity=off  Deterministic=off  OutPortSampleTime=sampleTimes.v2v
  Rate Transition1 : RateTransition  Integrity=off  Deterministic=off  OutPortSampleTime=sampleTimes.v2v
  Subsystem1 : Subsystem
  Sum : Sum  Inputs=++-
  Sum1 : Sum  Inputs=+-|
  Sum2 : Sum  Inputs=-|+
  Trigonometric Function : Trigonometry
  Wrap to Pi : Subsystem
  lateralError : Outport
  wires:
  Sum1/1 -> Wrap to Pi/1(In)
  Gain/1 -> Sum/3
  Product1/1 -> Gain/1
  targetCurvature/1 -> Product1/2
  Product/1 -> Add/2
  sensor/1 -> Rate Transition1/1
  Subsystem1/2(angle) -> Sum/1
  Wrap to Pi/1(Out) -> Sum/2
  Bus Selector2/1 -> Sum2/2, Sum1/1  "<heading>"
  Sum/1 -> Trigonometric Function/1
  Rate Transition/1 -> Bus Selector2/1
  Rate Transition1/1 -> Bus Selector1/1
  Add/1 -> lateralError/1
  Bus Selector1/1 -> Subsystem1/1(range)  "<range>"
  Bus Selector1/2 -> Subsystem1/2(azimuth)  "<azimuth>"
  Sum2/1 -> Subsystem1/3(dPsi)
  Bus Selector/2 -> Sum2/1  "<heading>"
  preceding/1 -> Bus Selector/1
  ego/1 -> Rate Transition/1
  Subsystem1/1(distance) -> Product1/1, Product/1
  Trigonometric Function/1 -> Product/2
  targetHeading/1 -> Sum1/2
  Bus Selector/1 -> Add/1  "<lateralError>"

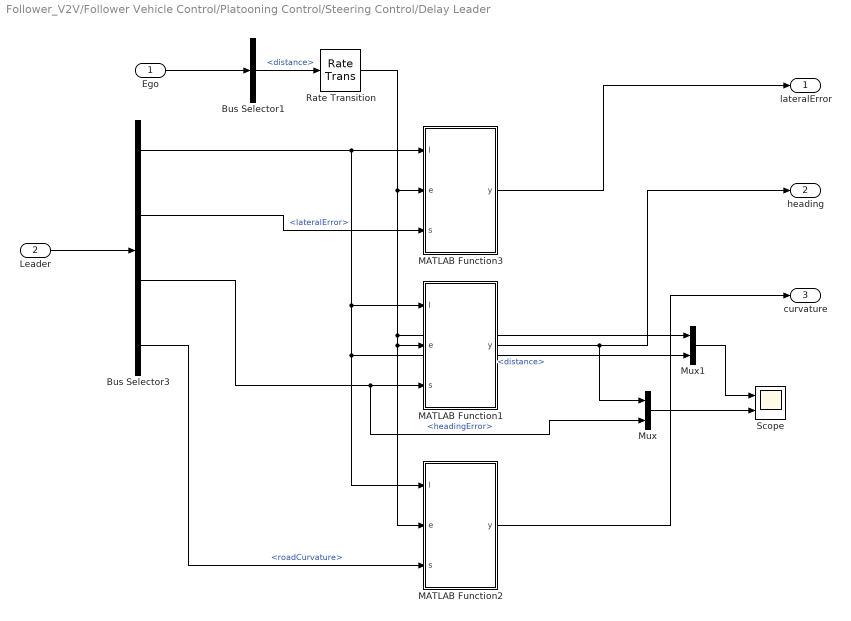
== system Follower_V2V/Follower Vehicle Control/Platooning Control/Steering Control/Delay Leader ==
  Ego : Inport
  Leader : Inport  Port=2
  Bus Selector1 : BusSelector  OutputSignals=distance
  Bus Selector3 : BusSelector  OutputSignals=distance,lateralError,headingError,roadCurvature
  MATLAB Function1 : MATLAB Function  TreatAsAtomicUnit=on
  MATLAB Function2 : MATLAB Function  TreatAsAtomicUnit=on
  MATLAB Function3 : MATLAB Function  TreatAsAtomicUnit=on
  Mux : Mux  Inputs=2
  Mux1 : Mux  Inputs=2
  Rate Transition : RateTransition  OutPortSampleTime=sampleTimes.v2v
  Scope : Scope  NumInputPorts=2
      settings: TimeRange=50.40000000000001  YMin=0~-5  YMax=12000~5  SaveName=ScopeData10
  lateralError : Outport
  heading : Outport  Port=2
  curvature : Outport  Port=3
  wires:
  MATLAB Function2/1(y) -> curvature/1
  Bus Selector3/4 -> MATLAB Function2/3(s)  "<roadCurvature>"
  MATLAB Function1/1(y) -> heading/1, Mux/1
  Bus Selector3/3 -> MATLAB Function1/3(s), Mux/2  "<headingError>"
  Mux1/1 -> Scope/1
  MATLAB Function3/1(y) -> lateralError/1
  Bus Selector3/2 -> MATLAB Function3/3(s)  "<lateralError>"
  Rate Transition/1 -> Mux1/1, MATLAB Function1/2(e), MATLAB Function2/2(e), MATLAB Function3/2(e)
  Bus Selector3/1 -> Mux1/2, MATLAB Function2/1(l), MATLAB Function1/1(l), MATLAB Function3/1(l)  "<distance>"
  Mux/1 -> Scope/2
  Bus Selector1/1 -> Rate Transition/1  "<distance>"
  Ego/1 -> Bus Selector1/1
  Leader/1 -> Bus Selector3/1

== system Follower_V2V/Follower Vehicle Control/Platooning Control/Steering Control/Remove initial spike ==
  In : Inport
  Compare To Constant : simulink/Logic and Bit Operations/Compare To Constant  relop=>  const=0.5  OutDataTypeStr=boolean
  Constant3 : Constant  Value=0
  Counter Free-Running : simulink/Sources/Counter Free-Running  NumBits=16  tsamp=-1
  Switch : Switch  Criteria=u2 > Threshold
  Weighted Sample Time Math : SampleTimeMath  TsampMathOp=*  weightValue=int32(1)  TsampMathImp=Offline Scaling Adjustment
  Out : Outport
  wires:
  In/1 -> Switch/1
  Switch/1 -> Out/1
  Counter Free-Running/1 -> Weighted Sample Time Math/1
  Weighted Sample Time Math/1 -> Compare To Constant/1
  Compare To Constant/1 -> Switch/2
  Constant3/1 -> Switch/3

== system Follower_V2V/Follower Vehicle Control/Platooning Control/Steering Control/Calculate lateral error/Subsystem1 ==
  range : Inport
  azimuth : Inport  Port=2
  dPsi : Inport  Port=3
  MATLAB Function : MATLAB Function  TreatAsAtomicUnit=on
  Wrap to Pi2 : Subsystem
  distance : Outport
  angle : Outport  Port=2
  wires:
  dPsi/1 -> Wrap to Pi2/1(In)
  azimuth/1 -> MATLAB Function/2(theta_c)
  MATLAB Function/2(theta) -> angle/1
  Wrap to Pi2/1(Out) -> MATLAB Function/3(dpsi)
  MATLAB Function/1(d) -> distance/1
  range/1 -> MATLAB Function/1(d_r)

== system Follower_V2V/Follower Vehicle Control/Platooning Control/Steering Control/Calculate lateral error/Wrap to Pi ==
  In : Inport
  Bias : Bias  Bias=pi
  Bias1 : Bias  Bias=-pi
  Constant : Constant  Value=2*pi
  Math Function : Math  Operator=mod  SaturateOnIntegerOverflow=on
  Out : Outport
  wires:
  In/1 -> Bias/1
  Bias/1 -> Math Function/1
  Math Function/1 -> Bias1/1
  Bias1/1 -> Out/1
  Constant/1 -> Math Function/2

== system Follower_V2V/Follower Vehicle Control/Platooning Control/Steering Control/Calculate lateral error/Subsystem1/Wrap to Pi2 ==
  In : Inport
  Bias : Bias  Bias=pi
  Bias1 : Bias  Bias=-pi
  Constant : Constant  Value=2*pi
  Math Function : Math  Operator=mod  SaturateOnIntegerOverflow=on
  Out : Outport
  wires:
  Constant/1 -> Math Function/2
  Bias1/1 -> Out/1
  Math Function/1 -> Bias1/1
  Bias/1 -> Math Function/1
  In/1 -> Bias/1

== matlab function Follower_V2V/Assignment/MATLAB Function ==
  data: dataIn input Bus: VehicleBus size=10; V2Vin input Bus: V2VBus size=10; myV2V input Bus: V2VBus size=1; brake input size=1; throttle input; gear input; clutch input; steering input; dataOut output Bus: VehicleBus size=10; vehicle input; V2Vout output Bus: V2VBus size=10
function [dataOut, V2Vout]  = fcn(dataIn, V2Vin, myV2V, brake,throttle,gear,clutch,steering, vehicle)
%#codegen

dataOut = dataIn;
dataOut(vehicle).control.brake = brake;
dataOut(vehicle).control.throttle = throttle;
dataOut(vehicle).control.clutch = clutch;
dataOut(vehicle).control.steering = steering;
dataOut(vehicle).control.gear = gear;

V2Vout = V2Vin;
V2Vout(vehicle) = myV2V;

== matlab function Follower_V2V/Selectors/MATLAB Function ==
  data: precedingTruth output Bus: VehicleBus size=1; egoTruth output Bus: VehicleBus size=1; leaderV2V output Bus: V2VBus size=1; data input Bus: VehicleBus size=10; V2V input Bus: V2VBus size=10; precedingV2V output Bus: V2VBus size=1; vehicle input
function [precedingTruth, egoTruth, leaderV2V, precedingV2V] = fcn(data, V2V, vehicle)
%#codegen

if (vehicle > 1)
    precedingTruth = data(vehicle-1);
    precedingV2V = V2V(vehicle-1);
else
    error('There is no preceeding vehicle!');
end
egoTruth = data(vehicle);

leaderV2V = V2V(1);

== stateflow chart Follower_V2V/Follower Vehicle Control/Enable Platooning ==
  state NotPlatooning
    en: platooning = logical(0);
    state GainSpeed
      en: headway = 1;
    state CloseDistance
      en: headway = 0.5;
    (default) -> GainSpeed
    GainSpeed -> CloseDistance : after(30,sec)[speed>10]
  state Platooning
    en: platooning = logical(1);
  (default) -> NotPlatooning
  CloseDistance -> Platooning : [prePlatooning && distance < 15]
  data: platooning output boolean; speed input; distance input; headway output; prePlatooning input boolean

== matlab function Follower_V2V/Follower Vehicle Control/Platooning Control/Steering Control/MATLAB Function ==
  data: a input; b input; c input; lambda input; V input; ydd_c output; ydd_p input; ydd_l input; eps input; epsd input; dy_l input; dv_l input
function ydd_c = fcn(a, b, c, lambda, V, ydd_p, ydd_l, eps, epsd,dy_l, dv_l)
%#codegen

if V < 1
    V = 1;
end

ydd_c = 1/(1+b)*(ydd_p + b*ydd_l - (a + lambda)*epsd/V^2 - a*lambda*eps/V^2 - (lambda*b+c)*dv_l/V^2 - lambda*c*dy_l/V^2);

== matlab function Follower_V2V/Follower Vehicle Control/Platooning Control/Steering Control/Calculate lateral error/Subsystem1/MATLAB Function ==
  data: d output; d_r input; theta_c input; theta output; dpsi input
function [d, theta] = fcn(d_r,theta_c,dpsi)
%#codegen

% Calculate distance and angle between centre of masses of two vehicles,
% assuming that theta_c is the angle measured from a camera (located lc
% distance ahead of the centre of mass of the follower vehicle) to the
% centre of the rear bumper of the preceding vehicle (a distance lb behind
% the centre of mass of the preceding vehicle, and that d is the distance
% measured from a radar sensor (located a distance lr ahead of the centre
% of mass of the following vehicle), to the same point on the bumper

lb = 2.5;   % Distance of rear bumper from CoM of preceding vehicle (estimated)
lr = 2.5;   % Distance of radar (distance sensor) from CoM of following vehicle (estimated)
lc = 1;     % Distance of camera (angle sensor) from CoM of following vehicle (estimated)

d_c = (lr -lc)*cos(theta_c) + sqrt(d_r^2 - (lr-lc)^2*sin(theta_c)^2);
theta_b = atan(d_c*sin(theta_c)/(d_c*cos(theta_c) + lc));

d_b = sqrt(d_c^2 + lc^2 + 2*d_c*lc*cos(theta_b));

d = sqrt(d_b^2 + lb^2 + 2*d_b*lb*cos(dpsi-theta_b));
theta = dpsi - atan((d_b*sin(dpsi-theta_b))/(d_b*cos(dpsi-theta_b)+lb));

== matlab function Follower_V2V/Data Models/Sensor Model/Radar Model/CG to Sensor transform/MATLAB Function ==
  data: d input; d_r output; theta input; dpsi input; theta_c output
function [d_r, theta_c] = fcn(d,theta,dpsi)
%#codegen

lb = 2.5;
lr = 2.5;
lc = 1;


A = d*sin(theta)/sin(pi-dpsi);
B = d*sin(dpsi-theta)/sin(pi-dpsi);

d_r = sqrt((A-lb)^2 + (B-lr)^2 - 2*(A-lb)*(B-lr)*cos(pi-dpsi));

d_c = sqrt((A-lb)^2 + (B-lc)^2 - 2*(A-lb)*(B-lc)*cos(pi-dpsi));

theta_c = asin(sin(pi-dpsi)*(A-lb)/d_c);

== matlab function Follower_V2V/Follower Vehicle Control/Platooning Control/Speed Control/MATLAB Function ==
  data: C1 input; d input; w input; xdd_p input; v_l input; xdd_c output; xdd_l input; eps input; epsd input; v input
function xdd_c = fcn(C1, d, w, xdd_p, v_l, xdd_l, eps, epsd, v)
%#codegen

% From Rajamani - Vehicle Dynamics and Control

xdd_c = (1-C1)*xdd_p + C1*xdd_l - (2*d - C1*(d + sqrt(d*d - 1)))*w*epsd ...
    - (d + sqrt(d*d - 1))*w*C1*(v-v_l) - w*w*eps;

== matlab function Follower_V2V/Follower Vehicle Control/Platooning Control/Steering Control/Curvature ==
  data: w input; V input; c output
function c = calcCurvature(w, V)
%#codegen

if V < 1
    V = 1;
end

c = w/V;

== matlab function Follower_V2V/Follower Vehicle Control/Platooning Control/Steering Control/Delay Leader/MATLAB Function1 ==
  data: l input; y output; e input; s input
function y = fcn(l,e,s)
%#codegen

n = 1000;
persistent S D;

if isempty(S)
    S = ones(n,1)*s;
    D = linspace(0.98*l,0.99*l,n);
end

D(1:(end-1)) = D(2:end);
D(end) = l;

S(1:(end-1)) = S(2:end);
S(end) = s;

[t i] = min(abs(D-e));

y = S(i);

== matlab function Follower_V2V/Follower Vehicle Control/Platooning Control/Steering Control/Delay Leader/MATLAB Function2 ==
  data: l input; y output; e input; s input
function y = fcn(l,e,s)
%#codegen

n = 1000;
persistent S D;

if isempty(S)
    S = ones(n,1)*s;
    D = linspace(0.98*l,0.99*l,n);
end

D(1:(end-1)) = D(2:end);
D(end) = l;

S(1:(end-1)) = S(2:end);
S(end) = s;

[t i] = min(abs(D-e));

y = S(i);

== matlab function Follower_V2V/Follower Vehicle Control/Platooning Control/Steering Control/Delay Leader/MATLAB Function3 ==
  data: l input; y output; e input; s input
function y = fcn(l,e,s)
%#codegen

n = 1000;
persistent S D;

if isempty(S)
    S = ones(n,1)*s;
    D = linspace(0.98*l,0.99*l,n);
end

D(1:(end-1)) = D(2:end);
D(end) = l;

S(1:(end-1)) = S(2:end);
S(end) = s;

[t i] = min(abs(D-e));

y = S(i);
